simulink model "DiscreteSystemStepResponse"  (R2019b)
settings: Solver=VariableStepAuto  StartTime=0.0  StopTime=15  RelTol=1e-6  AbsTol=1e-5
settings Model: Creator=19398  LastModifiedBy=19398

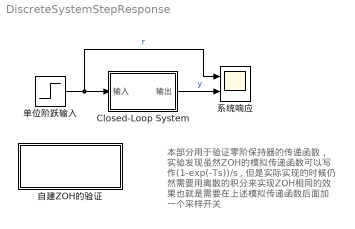
== system DiscreteSystemStepResponse ==
  note: 本部分用于验证零阶保持器的传递函数，
      | 实验发现虽然ZOH的模拟传递函数可以写
      | 作(1-exp(-Ts))/s，但是实际实现的时候仍
      | 然需要用离散的积分来实现ZOH相同的效
      | 果也就是需要在上述模拟传递函数后面加
      | 一个采样开关
  Closed-Loop System : Subsystem  mask{SampleTime=1}
      mask prompts: SampleTime "采样时间(s)"
  单位阶跃输入 : Step  SampleTime=0
  系统响应 : Scope  NumInputPorts=2
  自建ZOH的验证 : Subsystem
  wires:
  单位阶跃输入/1 -> Closed-Loop System/1(输入), 系统响应/1  "r"
  Closed-Loop System/1(输出) -> 系统响应/2  "y"

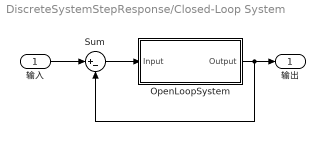
== system DiscreteSystemStepResponse/Closed-Loop System ==
  输入 : Inport
  OpenLoopSystem : Subsystem  mask{SampleTime=SampleTime}
      mask prompts: SampleTime "采样时间(s)"
  Sum : Sum  Inputs=|+-
  输出 : Outport
  wires:
  Sum/1 -> OpenLoopSystem/1(Input)
  OpenLoopSystem/1(Output) -> 输出/1, Sum/2
  输入/1 -> Sum/1

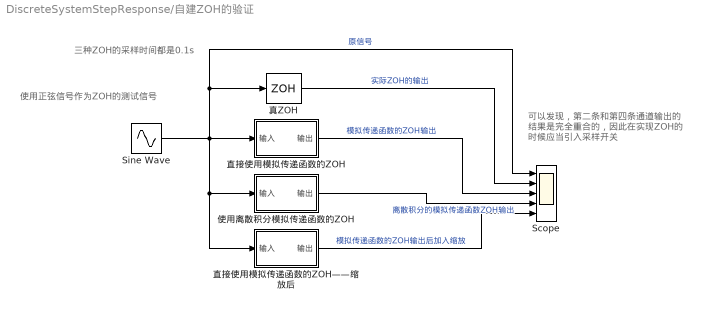
== system DiscreteSystemStepResponse/自建ZOH的验证 ==
  note: 可以发现，第二条和第四条通道输出的
      | 结果是完全重合的，因此在实现ZOH的
      | 时候应当引入采样开关
  note: 三种ZOH的采样时间都是0.1s
  note: 使用正弦信号作为ZOH的测试信号
  Scope : Scope  NumInputPorts=5
  Sine Wave : Sin  SampleTime=0
  使用离散积分模拟传递函数的ZOH : Subsystem
  直接使用模拟传递函数的ZOH : Subsystem
  直接使用模拟传递函数的ZOH——缩放后 : Subsystem
  真ZOH : ZeroOrderHold  SampleTime=0.1
  wires:
  Sine Wave/1 -> 直接使用模拟传递函数的ZOH——缩放后/1(输入), 使用离散积分模拟传递函数的ZOH/1(输入), 直接使用模拟传递函数的ZOH/1(输入), Scope/1, 真ZOH/1  "原信号"
  使用离散积分模拟传递函数的ZOH/1(输出) -> Scope/4  "离散积分的模拟传递函数ZOH输出"
  直接使用模拟传递函数的ZOH/1(输出) -> Scope/3  "模拟传递函数的ZOH输出"
  真ZOH/1 -> Scope/2  "实际ZOH的输出"
  直接使用模拟传递函数的ZOH——缩放后/1(输出) -> Scope/5  "模拟传递函数的ZOH输出后加入缩放"

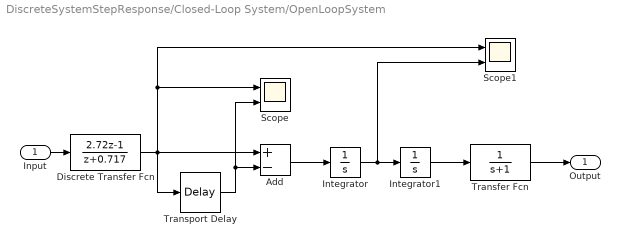
== system DiscreteSystemStepResponse/Closed-Loop System/OpenLoopSystem ==
  Input : Inport
  Add : Sum  Inputs=+-
  Discrete Transfer Fcn : DiscreteTransferFcn  Numerator=[2.72 -1]  Denominator=[1 0.717]  SampleTime=SampleTime
  Integrator : Integrator
  Integrator1 : Integrator
  Scope : Scope  NumInputPorts=2
  Scope1 : Scope  NumInputPorts=2
  Transfer Fcn : TransferFcn  Denominator=[1 1]
  Transport Delay : TransportDelay  DelayTime=SampleTime
  Output : Outport
  wires:
  Input/1 -> Discrete Transfer Fcn/1
  Integrator/1 -> Integrator1/1, Scope1/2
  Integrator1/1 -> Transfer Fcn/1
  Transfer Fcn/1 -> Output/1
  Add/1 -> Integrator/1
  Transport Delay/1 -> Scope/2, Add/2
  Discrete Transfer Fcn/1 -> Scope/1, Scope1/1, Add/1, Transport Delay/1

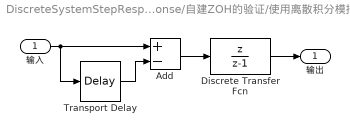
== system DiscreteSystemStepResponse/自建ZOH的验证/使用离散积分模拟传递函数的ZOH ==
  输入 : Inport
  Add : Sum  Inputs=+-
  Discrete Transfer Fcn : DiscreteTransferFcn  Numerator=[1 0]  Denominator=[1 -1]  SampleTime=0.1
  Transport Delay : TransportDelay  DelayTime=0.1
  输出 : Outport
  wires:
  Discrete Transfer Fcn/1 -> 输出/1
  Add/1 -> Discrete Transfer Fcn/1
  输入/1 -> Transport Delay/1, Add/1
  Transport Delay/1 -> Add/2

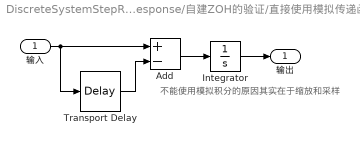
== system DiscreteSystemStepResponse/自建ZOH的验证/直接使用模拟传递函数的ZOH ==
  note: 不能使用模拟积分的原因其实在于缩放和采样
  输入 : Inport
  Add : Sum  Inputs=+-
  Integrator : Integrator
  Transport Delay : TransportDelay  DelayTime=0.1
  输出 : Outport
  wires:
  Integrator/1 -> 输出/1
  Add/1 -> Integrator/1
  输入/1 -> Transport Delay/1, Add/1
  Transport Delay/1 -> Add/2

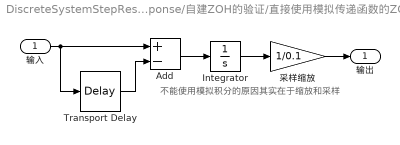
== system DiscreteSystemStepResponse/自建ZOH的验证/直接使用模拟传递函数的ZOH——缩放后 ==
  note: 不能使用模拟积分的原因其实在于缩放和采样
  输入 : Inport
  Add : Sum  Inputs=+-
  Integrator : Integrator
  Transport Delay : TransportDelay  DelayTime=0.1
  采样缩放 : Gain  Gain=1/0.1
  输出 : Outport
  wires:
  Integrator/1 -> 采样缩放/1
  Add/1 -> Integrator/1
  输入/1 -> Transport Delay/1, Add/1
  Transport Delay/1 -> Add/2
  采样缩放/1 -> 输出/1
